simulink model "Inverse_Kinematics"  (R2022b)
settings: Solver=VariableStepAuto  StartTime=0.0  StopTime=10.0  RelTol=1e-3
settings Model: Creator=sathwik  LastModifiedBy=sathwik

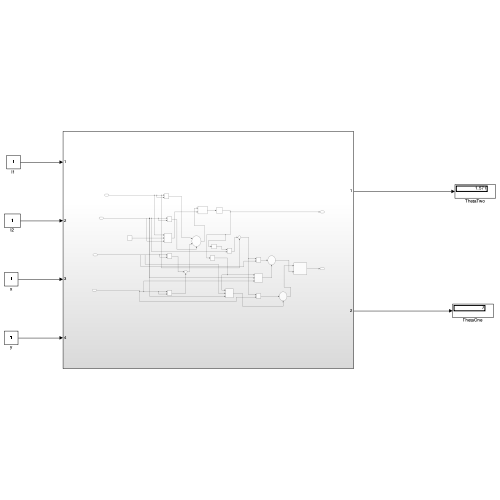
[thumbnail: Simulink's stored preview of the top-level diagram]
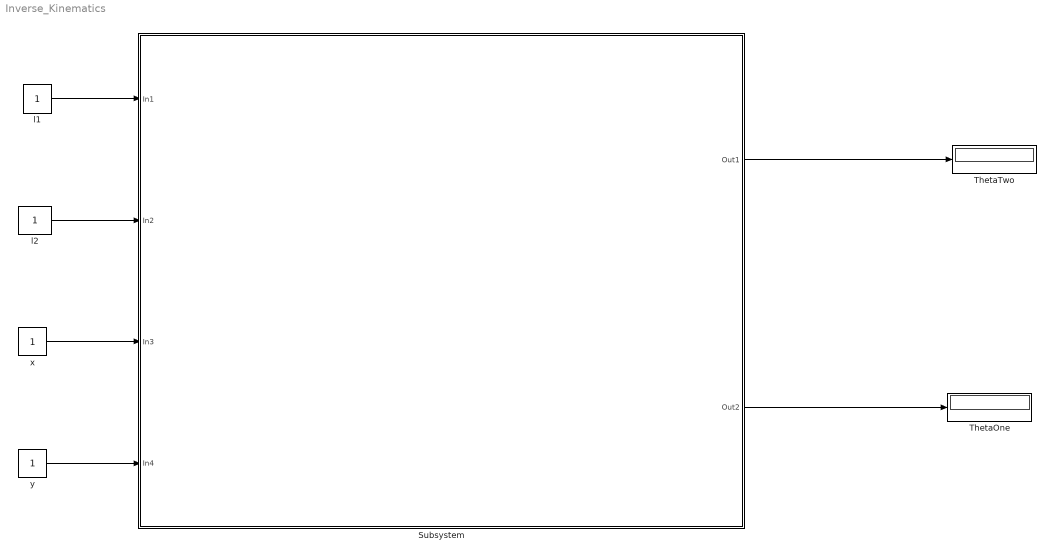
== system Inverse_Kinematics ==
  Subsystem : Subsystem
  ThetaOne : Display
  ThetaTwo : Display
  l1 : Constant
  l2 : Constant
  x : Constant
  y : Constant
  wires:
  l1/1 -> Subsystem/1(In1)
  l2/1 -> Subsystem/2(In2)
  x/1 -> Subsystem/3(In3)
  y/1 -> Subsystem/4(In4)
  Subsystem/1(Out1) -> ThetaTwo/1
  Subsystem/2(Out2) -> ThetaOne/1

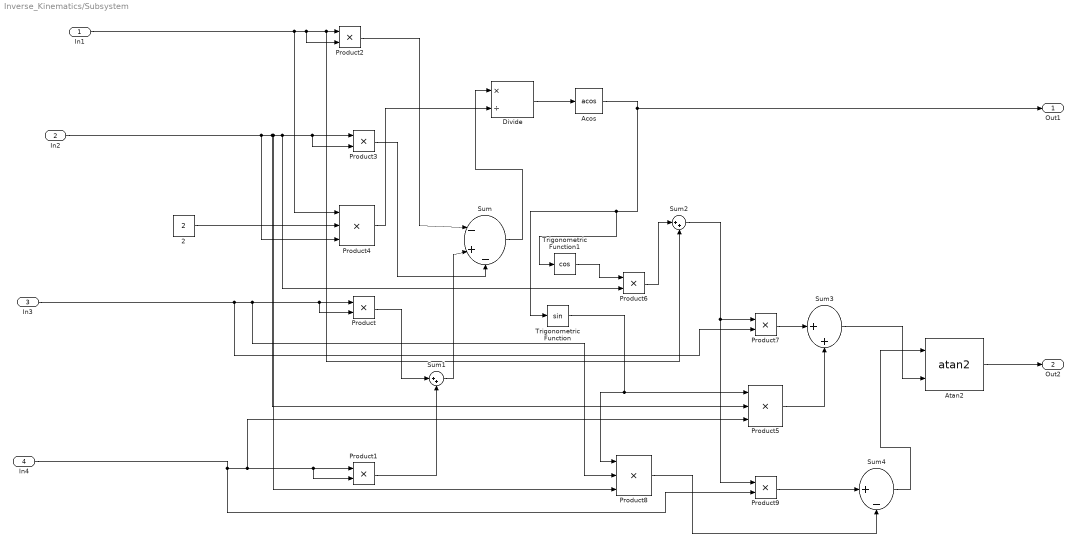
== system Inverse_Kinematics/Subsystem ==
  In1 : Inport
  In2 : Inport  Port=2
  In3 : Inport  Port=3
  In4 : Inport  Port=4
  2 : Constant  Value=2
  Acos : Trigonometry  Operator=acos
  Atan2 : Trigonometry  Operator=atan2
  Divide : Product  Inputs=*/
  Product{,1..3,6..7,9} (7 alike) : Product
  Product4 : Product  Inputs=3
  Product5 : Product  Inputs=3
  Product8 : Product  Inputs=3
  Sum : Sum  Inputs=|-+-
  Sum1 : Sum  Inputs=|++
  Sum2 : Sum  Inputs=|++
  Sum3 : Sum  Inputs=|++
  Sum4 : Sum  Inputs=|+-
  Trigonometric Function : Trigonometry
  Trigonometric Function1 : Trigonometry  Operator=cos
  Out1 : Outport
  Out2 : Outport  Port=2
  wires:
  Product8/1 -> Sum4/2
  Product4/1 -> Divide/2
  Product7/1 -> Sum3/1
  Atan2/1 -> Out2/1
  Sum/1 -> Divide/1
  In2/1 -> Product8/3, Product6/2, Product3/2, Product3/1, Product5/2, Product4/3
  Product5/1 -> Sum3/2
  Product2/1 -> Sum/1
  Product3/1 -> Sum/3
  Product6/1 -> Sum2/1
  In3/1 -> Product7/2, Product8/2, Product/2, Product/1
  In4/1 -> Product9/2, Product5/3, Product1/2, Product1/1
  Product/1 -> Sum1/1
  2/1 -> Product4/2
  Acos/1 -> Out1/1, Trigonometric Function1/1, Trigonometric Function/1
  Sum4/1 -> Atan2/1
  In1/1 -> Sum2/2, Product2/1, Product2/2, Product4/1
  Divide/1 -> Acos/1
  Sum1/1 -> Sum/2
  Sum2/1 -> Product9/1, Product7/1
  Sum3/1 -> Atan2/2
  Trigonometric Function1/1 -> Product6/1
  Product1/1 -> Sum1/2
  Product9/1 -> Sum4/1
  Trigonometric Function/1 -> Product8/1, Product5/1
